simulink model "ASM_Traffic_V2X_Complete_Model_2"  (R2019a)
settings: Solver=ode1  StartTime=SIM.tstart.v  StopTime=Inf  FixedStep=SIM.StepSize.v  RelTol=1e-3
PostLoadFcn:
  | if any(exist('dsrtsu_mdlpostloadfcn', 'file') ~= 0), dsrtsu_mdlpostloadfcn('Execute', bdroot); end
  | try, asm_mdl_postloadfcn(bdroot, 'UpdateModel', 2200); catch, disp(lasterr); end,
undefined symbols (not defined in the file): _SensorPnts_1, _SensorPnts_13, _SensorPnts_17, _SensorPnts_21, _SensorPnts_25, _SensorPnts_29, _SensorPnts_33, _SensorPnts_37, _SensorPnts_41, _SensorPnts_45, _SensorPnts_49, _SensorPnts_5, _SensorPnts_53, _SensorPnts_57, _SensorPnts_9, _to_, CPT, G5A, ITS, MDL, rad, s_to_rpm, SIM
libraries: simulink x169, ASM_VehicleDynamics_lib x126, ASM_Traffic_lib x83, ASM_Utils_lib x49, mdbs x45, ASM_Environment_lib x17, dspindex x12, dsaV2xLibraryAux x10, dsmpblib x6, dsaV2xAsn1Library x4, dsaV2xLibrary x4, ASM_BrakeHydraulics_lib x4
(part 2 of 36)

== system ASM_Traffic_V2X_Complete_Model_2/MDL/SoftECU ==
  Vehicle_Signals : Inport
  Environment_Signals : Inport  Port=2
  ASMSignalCollector : Subsystem
  Bus Creator : BusCreator  Inputs=4
  Bus Creator1 : BusCreator  Inputs=5
  Bus Creator2 : BusCreator  Inputs=5
  Bus Creator3 : BusCreator  Inputs=6
  Bus Creator4 : BusCreator  Inputs=4
  Bus Creator5 : BusCreator  Inputs=1
  Bus Creator6 : BusCreator  Inputs=5
  Bus Selector : BusSelector  OutputSignals=Drivetrain.Transmission.ActiveTransmission.Gear[],Environment.Driver.OutputSignals.Pos_AccPedal[%],Environment.Driver.OutputSignals.AutomaticTrmCtrlSignals.SelectorLever[-3T|-2P|-1R|0N|1D],Environment.Driver.OutputSignals.AutomaticTrmCtrlSignals.SW_TipTronic[-1Down|0Off|1Up]
  Bus Selector1 : BusSelector  OutputSignals=Maneuver.Parameters.Gear_Max[],Maneuver.MdlControl.Reset_VehicleStates[0|1],Maneuver.RefSignals.Gear_Maneuver[],Maneuver.ModeSignals.GearClutch_Mode[1Stim|2Driver|3OpenClutch|4RefGear]
  Bus Selector10 : BusSelector  OutputSignals=VehicleDynamics.Steering.SteeringWheelTorque.TrqSensor_Steering[Nm]
  Bus Selector11 : BusSelector  OutputSignals=BasicEngine.EngineTorques.Trq_Eff_Engine[Nm],VehicleDynamics.Brake.MasterBrakeCylinder.ActiveBrakeCylinder.p[bar],VehicleDynamics.VehicleMovement.Velocities.Vehicle.Linear.v_Vehicle_CoG[x;y;z][km|h].v_x_Vehicle_CoG[km|h],VehicleDynamics.VehicleMovement.Velocities.Vehicle.Linear.v_Vehicle_CoG[x;y;z][km|h].v_y_Vehicle_CoG[km|h],VehicleDynamics.VehicleMovement.Accelerations.VehicleCoG.Linear.a_Vehicle_CoG[x;y;z][m|s2].a_y_Vehicle_CoG[m|s2],VehicleDynamics.VehicleMovement.Velocities.Vehicle.Angular.w_Vehicle_CoG[x;y;z][deg|s].YawRate_Vehicle_CoG[deg|s],VehicleDynamics.Wheel.WheelSpeed,VehicleDynamics.Steering.Angle_SteeringWheel[deg],VehicleDynamics.Steering.i_Steering_Mean[],Environment.Driver.OutputSignals.Pos_AccPedal[%],Environment.Driver.OutputSignals.Pos_BrakePedal[%],VehicleDynamics.Suspension.SuspensionRear.SuspensionKinematicsRear.Kinematics_Left.Position_Left.Pos_RL_Wheel[x;y;z][m],VehicleDynamics.Suspension.SuspensionFront.RelativePositionFront.Pos_Wheel[FL;FR][x;y;z][m].Pos_FL_Wheel[x;y;z][m]
  Bus Selector12 : BusSelector  OutputSignals=Drivetrain.Crankshaft.n_Engine[rad|s],Drivetrain.Transmission.AutomaticTransmission.GearBox.omega_In_Trm[rad|s],Drivetrain.Transmission.ActiveTransmission.omega_Out_Trm[rad|s]
  Bus Selector13 : BusSelector  OutputSignals=VehicleDynamics.Brake.BrakeDisc.Const_BrakeDiscFactor
  Bus Selector14 : BusSelector  OutputSignals=VehicleDynamics.Tire.Tire_FL.ActiveTire.r_Dyn_FL_Tire[m],VehicleDynamics.Tire.Tire_RL.ActiveTire.r_Dyn_RL_Tire[m],VehicleDynamics.Tire.Tire_FR.ActiveTire.r_Dyn_FR_Tire[m],VehicleDynamics.Tire.Tire_RR.ActiveTire.r_Dyn_RR_Tire[m]  OutputAsBus=on
  Bus Selector15 : BusSelector  OutputSignals=Environment.Driver.OutputSignals.StartButtonSignals.Sw_StartButton[0Off|1On],Environment.Driver.OutputSignals.AutomaticTrmCtrlSignals.SelectorLever[-3T|-2P|-1R|0N|1D],Environment.Driver.OutputSignals.Pos_BrakePedal[%],Environment.Driver.OutputSignals.Pos_ClutchPedal[%]
  Bus Selector16 : BusSelector  OutputSignals=Sw_Ignition[0|1],Sw_StarterReq[0|1]
  Bus Selector17 : BusSelector  OutputSignals=State_Engine[0|1|2|3|4]
  Bus Selector18 : BusSelector  OutputSignals=Factor_Trq_Engine_Red[%]
  Bus Selector19 : BusSelector  OutputSignals=State_Engine[0|1|2|3|4]
  Bus Selector2 : BusSelector  OutputSignals=ESP_Trq_Intervention.Enable_TrqIncrease_ESP[0|1],ESP_Trq_Intervention.Trq_IncreaseRequest_ESP[Nm],ESP_Trq_Intervention.Enable_TrqDecrease_Fast_ESP[0|1],ESP_Trq_Intervention.Trq_DecreaseRequest_Fast_ESP[Nm],ESP_Trq_Intervention.Enable_TrqDecrease_Slow_ESP[0|1],ESP_Trq_Intervention.Trq_DecreaseRequest_Slow_ESP[Nm]
  Bus Selector20 : BusSelector  OutputSignals=Sw_Ignition[0|1]
  Bus Selector21 : BusSelector  OutputSignals=Maneuver.MdlControl.Reset_VehicleStates[0|1]
  Bus Selector3 : BusSelector  OutputSignals=Drivetrain.Crankshaft.n_Engine[rpm],BasicEngine.EngineTorques.Trq_Driver_Des[Nm],Environment.Driver.OutputSignals.Pos_AccPedal[%]
  Bus Selector4 : BusSelector  OutputSignals=Maneuver.MdlControl.Reset_VehicleStates[0|1]
  Bus Selector5 : BusSelector  OutputSignals=Enable_Trq_Increase_ACC[0|1],Trq_IncreaseRequest_ACC[Nm]
  Bus Selector6 : BusSelector  OutputSignals=VehicleDynamics.VehicleMovement.Velocities.Vehicle.Linear.v_Vehicle_CoG[x;y;z][km|h]
  Bus Selector7 : BusSelector  OutputSignals=Maneuver.MdlControl.Reset_VehicleStates[0|1],Maneuver.UserSignals_Customized.ECU_Commands[]
  Bus Selector8 : BusSelector  OutputSignals=Enable_Trq_Decrease_ACC[0|1],Trq_DecreaseRequest_ACC[Nm]
  Bus Selector9 : BusSelector  OutputSignals=Maneuver.MdlControl.Reset_VehicleStates[0|1]
  DisableReset : Subsystem
      mask Display: disp('DisableReset')
  Map_Inputs : Subsystem
  ModelDesk_MC_ID_SoftECU : ASM_Utils_lib/ModelDeskInterface/ModelDesk_MC_ID_SoftECU  Tag=ASM_MAINCOMPONENT  ASMProperties=struct('Name','SoftECU')
  OpenBrkHydModel : Subsystem
      settings: OpenFcn=asm_open_lib('ASM_BrakeHydraulics_lib/Demos');
      mask Display: disp('Open\nASM_Brakehydraulics_lib')
  SOFT_ECU_POWERSTEERING : ASM_VehicleDynamics_lib/SoftECU/SoftECU_Steering/SOFT_ECU_POWERSTEERING  Tag=ASM_SUBCOMPONENT  Const_t_PowerSteering=MDL.SoftECU.SoftECUPowerSteering.Const_t_PowerSteering  Map_Trq_PowerSteering=MDL.SoftECU.SoftECUPowerSteering.Map_Trq_PowerSteering  StepSize=SIM.StepSize  ASMProperties=struct('Name','SOFT_ECU_POWERSTEERING','Version','3.0','Library','ASM_VehicleDynamics_lib')  ASMInstanceName=soft_ecu_powersteering  ASMInstanceID=1
  START_BUTTON : ASM_VehicleDynamics_lib/SoftECU/SoftECU_Body/START_BUTTON  Tag=ASM_SUBCOMPONENT  Const_t_Min_Active=MDL.SoftECU.StartButton.Const_t_Min_Active  Const_t_Min_Starter=MDL.SoftECU.StartButton.Const_t_Min_Starter  Const_Post_ClutchPedal_LowLim=MDL.SoftECU.StartButton.Const_Post_ClutchPedal_LowLim  Const_Post_BrakePedal_LowLim=MDL.SoftECU.StartButton.Const_Post_BrakePedal_LowLim  StepSize=SIM.StepSize  ASMProperties=struct('Name','START_BUTTON','Version','1.0','Library','ASM_VehicleDynamics_lib')  ASMInstanceName=start_button  ASMInstanceID=1
  Soft_ECU_ACC : Subsystem
  Soft_ECU_Brake : Subsystem  Tag=ASM_SOFT_ECU_BRAKE
      settings: AttributesFormatString=BASIC
  Soft_ECU_Engine_Basic : Subsystem
  Soft_ECU_Transmission : Subsystem
  StarterPermanentOn_Handling : Subsystem
  SoftECU_Signals : Outport
  tag scope: ASMBUS_SoftECU_ACC=global, ASMBUS_SoftECU_Brake=global, ASMBUS_SoftECU_Engine=global, ASMBUS_SoftECU_PowerSteering=global, ASMBUS_SoftECU_StartButton=global, ASMBUS_SoftECU_Transmission=global
  wires:
  DisableReset/1(Reset[0|1]) -> START_BUTTON/10
  Bus Selector21/1 -> DisableReset/1(Reset_VehicleStates[0|1])  "<Reset_VehicleStates[0|1]>"
  Bus Selector20/1 -> SOFT_ECU_POWERSTEERING/4  "<Sw_Ignition[0|1]>"
  Bus Selector19/1 -> Soft_ECU_Transmission/4(State_Engine[0|1|2|3|4])  "<State_Engine[0|1|2|3|4]>"
  [TAG_FromIO_Engine] -> Bus Selector17/1, Bus Selector19/1
  [TAG_FromIO_Drivetrain] -> Bus Selector18/1
  Bus Selector18/1 -> Soft_ECU_Engine_Basic/15(Factor_Trq_Engine_Red[%])  "<Factor_Trq_Engine_Red[%]>"
  Bus Selector16/2 -> Soft_ECU_Engine_Basic/5(Sw_StarterReq[0Off|1On])  "<Sw_StarterReq[0|1]>"
  Bus Selector16/1 -> Soft_ECU_Engine_Basic/4(Sw_Ignition[0Off|1On])  "<Sw_Ignition[0|1]>"
  [TAG_FromIO_Body] -> Bus Selector16/1, Bus Selector20/1
  START_BUTTON/1 -> [ASMBUS_SoftECU_StartButton]
  Bus Selector15/1 -> START_BUTTON/5  "<Sw_StartButton[0Off|1On]>"
  Bus Selector15/2 -> START_BUTTON/6  "<SelectorLever[-3T|-2P|-1R|0N|1D]>"
  Bus Selector15/3 -> START_BUTTON/7  "<Pos_BrakePedal[%]>"
  Bus Selector15/4 -> START_BUTTON/8  "<Pos_ClutchPedal[%]>"
  START_BUTTON/2 -> Bus Creator1/1  "State_StartButton[-2|-1|0|1|2|3]"
  START_BUTTON/6 -> Bus Creator1/5  "Sw_StarterReq[0|1]"
  START_BUTTON/3 -> Bus Creator1/2  "Lock[0|1]"
  START_BUTTON/4 -> Bus Creator1/3  "Sw_Acc[0|1]"
  START_BUTTON/5 -> Bus Creator1/4  "Sw_Ignition[0|1]"
  Bus Creator1/1 -> Bus Creator3/6  "ECU_Body"
  [TAG_Sw_Transmission_Mode] -> START_BUTTON/1
  [TAG_SoftECU_State_KeyFob] -> START_BUTTON/2
  Bus Selector17/1 -> START_BUTTON/9  "<State_Engine[0|1|2|3|4]>"
  StarterPermanentOn_Handling/1(State_StartButton_Ext[-1|0|1|2]) -> START_BUTTON/3
  StarterPermanentOn_Handling/2(Mode_StartButtonState[1Stim|2SoftECU]) -> START_BUTTON/4
  Bus Selector12/3 -> Soft_ECU_Transmission/3(omega_Out_Trm[rad|s])  "<omega_Out_Trm[rad|s]>"
  Bus Selector12/2 -> Soft_ECU_Transmission/2(omega_In_Trm[rad|s])  "<omega_In_Trm[rad|s]>"
  Bus Selector12/1 -> Soft_ECU_Transmission/1(n_Engine[rad|s])  "<n_Engine[rad|s]>"
  [TAG_SoftECU_ESP_Switches] -> Map_Inputs/3(Switches_ESP_User)
  Bus Selector7/2 -> Map_Inputs/2(ECU_Commands[])  "<ECU_Commands[]>"
  Map_Inputs/2(Sw_ASR[0Off|1On]) -> Soft_ECU_Brake/7(Sw_ASR[0Off|1On])
  Map_Inputs/1(Sw_ESP[0Off|1ABS|ESP]) -> Soft_ECU_Brake/6(Sw_ESP[0Off|1ABS|2ESP])
  Soft_ECU_Brake/1(ASMSignalBus) -> [ASMBUS_SoftECU_Brake]
  Soft_ECU_Brake/6(Trq_Intervention) -> Bus Creator6/5
  Soft_ECU_Brake/5(Valves) -> Bus Creator6/4
  Soft_ECU_Brake/4(ECU_Mode[0None|1ABS|2ESP|3ASR]) -> Bus Creator6/3
  Soft_ECU_Brake/3(p_Brake_Desired[bar]) -> Bus Creator6/2
  Soft_ECU_Brake/2(Enable_p_Brake_Desired[0|1]) -> Bus Creator6/1
  Bus Selector14/1 -> Soft_ECU_Brake/21(r_Tire[m])
  Bus Selector11/13 -> Soft_ECU_Brake/20(Pos_FL_Wheel[x;y;z][m])  "<Pos_FL_Wheel[x;y;z][m]>"
  Bus Selector11/12 -> Soft_ECU_Brake/19(Pos_RL_Wheel[x;y;z][m])  "<Pos_RL_Wheel[x;y;z][m]>"
  Bus Selector11/11 -> Soft_ECU_Brake/18(Pos_BrakePedal[%])  "<Pos_BrakePedal[%]>"
  Bus Selector11/10 -> Soft_ECU_Brake/17(Pos_AccPedal[%])  "<Pos_AccPedal[%]>"
  Bus Selector11/2 -> Soft_ECU_Brake/9(p_MasterBrakeCyl[bar])  "<p[bar]>"
  Bus Selector11/3 -> Soft_ECU_Brake/10(v_x_Vehicle_CoG[km|h])  "<v_x_Vehicle_CoG[km|h]>"
  Bus Selector11/4 -> Soft_ECU_Brake/11(v_y_Vehicle_CoG[km|h])  "<v_y_Vehicle_CoG[km|h]>"
  Bus Selector11/5 -> Soft_ECU_Brake/12(a_y_Vehicle_CoG[m|s2])  "<a_y_Vehicle_CoG[m|s2]>"
  Bus Selector11/6 -> Soft_ECU_Brake/13(YawRate_Vehicle_CoG[deg|s])  "<YawRate_Vehicle_CoG[deg|s]>"
  Bus Selector11/7 -> Soft_ECU_Brake/14(WheelSpeed[FL;FR;RL;RR][rad|s])  "<WheelSpeed>"
  Bus Selector11/8 -> Soft_ECU_Brake/15(Angle_SteeringWheel[deg])  "<Angle_SteeringWheel[deg]>"
  Bus Selector11/9 -> Soft_ECU_Brake/16(i_Steering_Mean[])  "<i_Steering_Mean[]>"
  Bus Selector11/1 -> Soft_ECU_Brake/8(Trq_Eff_Engine[Nm])  "<Trq_Eff_Engine[Nm]>"
  Bus Selector7/1 -> Soft_ECU_Brake/5(Reset[]), Map_Inputs/1(Reset[0|1])  "<Reset_VehicleStates[0|1]>"
  Bus Selector13/1 -> Soft_ECU_Brake/4(Const_BrakeDiscFactor[FL;FR;RL;RR][m3])  "<Const_BrakeDiscFactor>"
  Bus Selector9/1 -> SOFT_ECU_POWERSTEERING/2  "<Reset_VehicleStates[0|1]>"
  Bus Selector10/1 -> SOFT_ECU_POWERSTEERING/1  "<TrqSensor_Steering[Nm]>"
  Bus Selector/2 -> Soft_ECU_Transmission/6(Pos_AccPedal_Driver[%])  "<Pos_AccPedal[%]>"
  Bus Selector/3 -> Soft_ECU_Transmission/7(SelectorLever[-3T|-2P|-1R|0N|1D])  "<SelectorLever[-3T|-2P|-1R|0N|1D]>"
  Bus Selector/4 -> Soft_ECU_Transmission/8(TipShift[-1Down|0Off|1Up])  "<SW_TipTronic[-1Down|0Off|1Up]>"
  Bus Selector3/3 -> Soft_ECU_Engine_Basic/3(Pos_AccPedal_Driver[%])  "<Pos_AccPedal[%]>"
  Bus Selector8/2 -> Soft_ECU_Brake/3(Trq_Request_Extern[Nm])  "<Trq_DecreaseRequest_ACC[Nm]>"
  Bus Selector8/1 -> Soft_ECU_Brake/2(Enable_Trq_Extern[0|1]), Soft_ECU_Brake/1(State_Brake_Without_BrkPedal[0|1])  "<Enable_Trq_Decrease_ACC[0|1]>"
  Bus Selector1/2 -> Soft_ECU_Transmission/10(Reset[0|1])  "<Reset_VehicleStates[0|1]>"
  Bus Selector1/1 -> Soft_ECU_Transmission/9(Gear_Max_Maneuver[0Off|1_n])  "<Gear_Max[]>"
  Soft_ECU_Transmission/5(Gear[]) -> Bus Creator/4  "Gear[]"
  Soft_ECU_Transmission/4(Ctrl_Lockup_Clutch[%]) -> Bus Creator/3  "Ctrl_Lockup_Clutch[%]"
  Soft_ECU_Transmission/3(Ctrl_Parking_Pawl[0|1]) -> Bus Creator/2  "Ctrl_Parking_Pawl[0|1]"
  Soft_ECU_Transmission/1(ASMSignalBus) -> [ASMBUS_SoftECU_Transmission]
  Soft_ECU_Transmission/2(Factor_Trq_Engine_Red[%]) -> Bus Creator/1  "Factor_Trq_Engine_Red[%]"
  Bus Selector/1 -> Soft_ECU_Transmission/5(Gear_Current[])  "<Gear[]>"
  Bus Selector1/3 -> Soft_ECU_Transmission/11(Gear_Maneuver[])  "<Gear_Maneuver[]>"
  Bus Selector1/4 -> Soft_ECU_Transmission/12(GearClutch_Mode[1Stim|2SoftECU|3OpenClutch|4RefGear])  "<GearClutch_Mode[1Stim|2Driver|3OpenClutch|4RefGear]>"
  Bus Selector4/1 -> Soft_ECU_Engine_Basic/6(Reset[])  "<Reset_VehicleStates[0|1]>"
  Bus Selector3/1 -> Soft_ECU_Engine_Basic/1(n_Engine[rpm])  "<n_Engine[rpm]>"
  Bus Selector3/2 -> Soft_ECU_Engine_Basic/2(Trq_Driver_Des[Nm])  "<Trq_Driver_Des[Nm]>"
  Soft_ECU_Engine_Basic/2(Engine_Dynamic_Fast[0|1]) -> Bus Creator2/1  "Engine_Dynamic_Fast[0|1]"
  Soft_ECU_Engine_Basic/3(Pos_AccPedal_Influenced[%]) -> Bus Creator2/2  "Pos_AccPedal_Influenced[%]"
  Soft_ECU_Engine_Basic/4(Pos_AccPedal_Driver_Des[%]) -> Bus Creator2/3  "Pos_AccPedal_Driver_Des[%]"
  Bus Creator2/1 -> Bus Creator3/1  "ECU_Engine"
  Soft_ECU_Engine_Basic/1(ASMSignalBus) -> [ASMBUS_SoftECU_Engine]
  Soft_ECU_Engine_Basic/5(Sw_Starter[0Off|1On]) -> Bus Creator2/4  "Sw_Starter[0Off|1On]"
  Soft_ECU_Engine_Basic/6(State_Engine[0|1|2|3|4]) -> Bus Creator2/5  "State_Engine[0|1|2|3|4]"
  Bus Creator5/1 -> Bus Creator3/5  "ECU_PowerSteering"
  SOFT_ECU_POWERSTEERING/2 -> Bus Creator5/1  "Trq_PowerSteering[Nm]"
  Bus Selector6/1 -> SOFT_ECU_POWERSTEERING/3  "<v_Vehicle_CoG[x;y;z][km|h]>"
  SOFT_ECU_POWERSTEERING/1 -> [ASMBUS_SoftECU_PowerSteering]
  [TAG_FromIO_Brake] -> Bus Selector2/1
  Bus Selector2/1 -> Soft_ECU_Engine_Basic/7(Enable_TrqIncrease_Fast_ESP[0|1])  "<Enable_TrqIncrease_ESP[0|1]>"
  Bus Selector2/2 -> Soft_ECU_Engine_Basic/8(Trq_IncreaseRequest_Fast_ESP[Nm])  "<Trq_IncreaseRequest_ESP[Nm]>"
  Bus Selector2/3 -> Soft_ECU_Engine_Basic/9(Enable_TrqDecrease_Fast_ESP[0|1])  "<Enable_TrqDecrease_Fast_ESP[0|1]>"
  Bus Selector2/4 -> Soft_ECU_Engine_Basic/10(Trq_DecreaseRequest_Fast_ESP[Nm])  "<Trq_DecreaseRequest_Fast_ESP[Nm]>"
  Bus Selector2/5 -> Soft_ECU_Engine_Basic/11(Enable_TrqDecrease_Slow_ESP[0|1])  "<Enable_TrqDecrease_Slow_ESP[0|1]>"
  Bus Selector2/6 -> Soft_ECU_Engine_Basic/12(Trq_DecreaseRequest_Slow_ESP[Nm])  "<Trq_DecreaseRequest_Slow_ESP[Nm]>"
  Soft_ECU_ACC/2(Enable_Trq_Engine_ACC[0|1]) -> Bus Creator4/1  "Enable_Trq_Increase_ACC[0|1]"
  Soft_ECU_ACC/3(Trq_Request_Engine_ACC[Nm]) -> Bus Creator4/2  "Trq_IncreaseRequest_ACC[Nm]"
  Soft_ECU_ACC/4(Enable_Trq_Brake_ACC[0|1]) -> Bus Creator4/3  "Enable_Trq_Decrease_ACC[0|1]"
  Soft_ECU_ACC/5(Trq_Request_Brake_ACC[Nm]) -> Bus Creator4/4  "Trq_DecreaseRequest_ACC[Nm]"
  Bus Creator3/1 -> SoftECU_Signals/1  "SoftECU"
  Bus Creator6/1 -> Bus Creator3/3  "ECU_Brake"
  Bus Creator4/1 -> Bus Creator3/4  "ECU_ACC"
  Bus Creator/1 -> Bus Creator3/2  "ECU_Transmission"
  [TAG_FromIO_ACC] -> Bus Selector5/1, Bus Selector8/1
  Bus Selector5/1 -> Soft_ECU_Engine_Basic/13(Enable_Trq_Extern[0|1])  "<Enable_Trq_Increase_ACC[0|1]>"
  Bus Selector5/2 -> Soft_ECU_Engine_Basic/14(Trq_Request_Extern[Nm])  "<Trq_IncreaseRequest_ACC[Nm]>"
  Soft_ECU_ACC/1(ASMSignalBus) -> [ASMBUS_SoftECU_ACC]
  Vehicle_Signals/1 -> Bus Selector3/1, Bus Selector12/1, Bus Selector/1, Bus Selector13/1, Bus Selector11/1, Bus Selector14/1, Soft_ECU_ACC/2(Vehicle_Signals), Bus Selector10/1, Bus Selector6/1, Bus Selector15/1
  Environment_Signals/1 -> Bus Selector4/1, Bus Selector1/1, Bus Selector7/1, Soft_ECU_ACC/1(Environment_Signals), Bus Selector9/1, Bus Selector21/1

== system ASM_Traffic_V2X_Complete_Model_2/MDL/VehicleDynamics ==
  Trq_Shaft[FL,FR,RL,RR][Nm] : Inport
  Environment_Signals : Inport  Port=2
  AERODYNAMICS : ASM_VehicleDynamics_lib/VehicleDynamics/Aerodynamics/AERODYNAMICS  Tag=ASM_SUBCOMPONENT  Map_C_x=MDL.VehicleDynamics.Aerodynamics.Map_C_x  Map_C_y=MDL.VehicleDynamics.Aerodynamics.Map_C_y  Map_C_z=MDL.VehicleDynamics.Aerodynamics.Map_C_z  Map_C_M_x=MDL.VehicleDynamics.Aerodynamics.Map_C_M_x  Map_C_M_y=MDL.VehicleDynamics.Aerodynamics.Map_C_M_y  Map_C_M_z=MDL.VehicleDynamics.Aerodynamics.Map_C_M_z  Const_A_x=MDL.VehicleDynamics.Aerodynamics.Const_A_x  Const_PosVec_VtoRefAero=MDL.VehicleDynamics.Aerodynamics.Const_PosVec_RefAero_CoorSysV  Const_Char_Length=MDL.VehicleDynamics.Aerodynamics.Const_Char_Length  Const_Dens_Air=MDL.VehicleDynamics.Aerodynamics.Const_Dens_Air  ASMProperties=struct('Name','AERODYNAMICS','Version','5.0','Library','ASM_VehicleDynamics_lib')  ASMInstanceName=aerodynamics  ASMInstanceID=1
  ASMSignalCollector : Subsystem
  Brake : Subsystem
  Bus Selector1 : BusSelector  OutputSignals=Road.Road_ContactPoints.Sw_Tire_Parameter_Set_CP[FL;FR;RL;RR][1|2|3|4],Road.Road_ContactPoints.Fric_Coeff_CP[FL;FR;RL;RR][],Road.Road_ContactPoints.Pos_z_CP[FL;FR;RL;RR][m],Road.Road_ContactPoints.UnitVec_z_CP[FL;FR;RL;RR][x;y;z],Road.Road_InitialStates.Pos_Vehicle_Init_CoorSys_E[x;y;z][m],Road.Road_InitialStates.Angle_Vehicle_Init_CoorSys_E[x;y;z][rad],Maneuver.MdlControl.Reset_VehicleStates[0|1],Maneuver.MdlControl.Keep_VehiclePosition[0|1],Driver.Pos_BrakePedal[%],Driver.Angle_SteeringWheel[deg],Road.Road_ASMVeh.v_Wind_Coor_Sys_E[x;y;z][m|s],Road.Ambient.p_Ambient[Pa],Driver.ParkingBrakeSignals.Sw_ParkingBrake[0Off|1On],Road.Ambient.T_Ambient[degC],Driver.Pos_AccPedal[%],Maneuver.VehicleInitStates.q_dt_Vehicle_Init[6x1],Maneuver.RefSignals.Trq_Steering_Maneuver[Nm],Maneuver.RefSignals.Sw_SteeringMode_Maneuver[1Angle|2Trq]
  Bus Selector2 : BusSelector  OutputSignals=w_Rel_FL_Wheel_dDispl_SteeringRod_dt[x;y;z][rad|m],w_Rel_FR_Wheel_dDispl_SteeringRod_dt[x;y;z][rad|m]  OutputAsBus=on
  Bus Selector3 : BusSelector  OutputSignals=Pos_FL_Wheel_dDispl_SteeringRod[x;y;z][],Pos_FR_Wheel_dDispl_SteeringRod[x;y;z][]  OutputAsBus=on
  Bus Selector4 : BusSelector  OutputSignals=Trq_PowerSteering[Nm]  OutputAsBus=on
  Bus Selector5 : BusSelector  OutputSignals=EPSMotorStates_External[Angle;Angle_dt][rad;rad|s]  OutputAsBus=on
  CommonVehicleParameters : Subsystem
      settings: CopyFcn=|
      | try
      |  set_param(gcb,'LinkStatus', 'none')
      | catch
      | end
      mask Display: disp('Common vehicle parameters')
  Constant : Constant  Value=0
  DerivativeAddition : Subsystem
  F_External_CoorSys_V[x,y,z][N] : Constant  Value=[0 0 0]
  ModelDesk_MC_ID_VehicleDynamics : ASM_Utils_lib/ModelDeskInterface/ModelDesk_MC_ID_VehicleDynamics  Tag=ASM_MAINCOMPONENT  ASMProperties=struct('Name','VehicleDynamics')
  OR : Subsystem
  STEERING_3DOF_VARIABLE_RATIO : ASM_VehicleDynamics_lib/VehicleDynamics/Steering/STEERING_3DOF_VARIABLE_RATIO  Tag=ASM_SUBCOMPONENT  SW_EPSLocation=MDL.VehicleDynamics.Steering3DOF.SW_EPSLocation  SW_EPSSimulation=MDL.VehicleDynamics.Steering3DOF.SW_EPSSimulation  SW_ExternalEPSOutput=MDL.VehicleDynamics.Steering3DOF.SW_ExternalEPSOutput  SW_LocationColumnStiffness=MDL.VehicleDynamics.Steering3DOF.SW_LocationColumnStiffness  SW_DriverHand=MDL.VehicleDynamics.Steering3DOF.SW_DriverHand  Map_i_Steering=MDL.VehicleDynamics.Steering3DOF.Map_i_Steering  Const_i_EPSSteeringColumn=MDL.VehicleDynamics.Steering3DOF.Const_i_EPSSteeringColumn  Const_i_EPSSteeringRod=MDL.VehicleDynamics.Steering3DOF.Const_i_EPSSteeringRod  Const_Angle_Max_SteeringWheel=MDL.VehicleDynamics.Steering3DOF.Const_Angle_Max_SteeringWheel  Const_CardanAngle_UpperJoint=MDL.VehicleDynamics.Steering3DOF.Const_CardanAngle_UpperJoint  Const_CardanAngle_LowerJoint=MDL.VehicleDynamics.Steering3DOF.Const_CardanAngle_LowerJoint  Const_AngleOffsetCardanJoints=MDL.VehicleDynamics.Steering3DOF.Const_InitialAngle_LowerCardanJoint  Const_InitialAngle_UpperCardanJoint=MDL.VehicleDynamics.Steering3DOF.Const_InitialAngle_UpperCardanJoint  Const_MaxTorque_Driver=MDL.VehicleDynamics.Steering3DOF.Const_MaxTorque_Driver  Const_Inertia_SteeringWheel=MDL.VehicleDynamics.Steering3DOF.Const_Inertia_SteeringWheel  Const_Inertia_LowerSteeringColumn=MDL.VehicleDynamics.Steering3DOF.Const_Inertia_LowerSteeringColumn  SW_SteeringColumn_Stiffness=MDL.VehicleDynamics.Steering3DOF.SW_SteeringColumn_Stiffness  Map_TrqSpring_SteeringColumn=MDL.VehicleDynamics.Steering3DOF.Map_TrqSpring_SteeringColumn  Const_Stiffness_SteeringColumn=MDL.VehicleDynamics.Steering3DOF.Const_Stiffness_SteeringColumn  Const_Damping_SteeringColumn=MDL.VehicleDynamics.Steering3DOF.Const_Damping_SteeringColumn  Const_Time_SteeringWheel=MDL.VehicleDynamics.Steering3DOF.Const_Time_SteeringWheel  Const_Stiffness_DriverHand=MDL.VehicleDynamics.Steering3DOF.Const_Stiffness_DriverHand  Const_Damping_DriverHand=MDL.VehicleDynamics.Steering3DOF.Const_Damping_DriverHand  Const_Inertia_EPS=MDL.VehicleDynamics.Steering3DOF.Const_Inertia_EPS  Const_Stiffness_EPS=MDL.VehicleDynamics.Steering3DOF.Const_Stiffness_EPS  Const_Damping_EPS=MDL.VehicleDynamics.Steering3DOF.Const_Damping_EPS  Const_Damping_LowerSteeringColumn=MDL.VehicleDynamics.Steering3DOF.Const_Damping_LowerSteeringColumn  SW_SF_SteeringWheel=MDL.VehicleDynamics.Steering3DOF.SpringFriction.SW_SF_SteeringWheel  Const_Stiffness_SF_SteeringWheel=MDL.VehicleDynamics.Steering3DOF.SpringFriction.Const_Stiffness_SF_SteeringWheel  Const_LimitingTorque_SF_SteeringWheel=MDL.VehicleDynamics.Steering3DOF.SpringFriction.Const_LimitingTorque_SF_SteeringWheel  SW_ESF_SteeringWheel=MDL.VehicleDynamics.Steering3DOF.ExponentialSpringFriction.SW_ESF_SteeringWheel  Const_Stiffness_ESF_SteeringWheel=MDL.VehicleDynamics.Steering3DOF.ExponentialSpringFriction.Const_Stiffness_ESF_SteeringWheel  Const_LimitingTorque_ESF_SteeringWheel=MDL.VehicleDynamics.Steering3DOF.ExponentialSpringFriction.Const_LimitingTorque_ESF_SteeringWheel  SW_CF_SteeringRod=MDL.VehicleDynamics.Steering3DOF.CoulombFriction.SW_CF_SteeringRod  Const_LimitingForce_CF_SteeringRod=MDL.VehicleDynamics.Steering3DOF.CoulombFriction.Const_LimitingForce_CF_SteeringRod  Const_Damping_CF_SteeringRod=MDL.VehicleDynamics.Steering3DOF.CoulombFriction.Const_Damping_CF_SteeringRod  SW_MF_SteeringRod=MDL.VehicleDynamics.Steering3DOF.MaxwellFriction.SW_MF_SteeringRod  Const_Stiffness_MF_SteeringRod=MDL.VehicleDynamics.Steering3DOF.MaxwellFriction.Const_Stiffness_MF_SteeringRod  Const_LimitingForce_MF_SteeringRod=MDL.VehicleDynamics.Steering3DOF.MaxwellFriction.Const_LimitingForce_MF_SteeringRod  Const_Damping_MF_SteeringRod=MDL.VehicleDynamics.Steering3DOF.MaxwellFriction.Const_Damping_MF_SteeringRod  SW_SF_SteeringRod=MDL.VehicleDynamics.Steering3DOF.SpringFriction.SW_SF_SteeringRod  Const_Stiffness_SF_SteeringRod=MDL.VehicleDynamics.Steering3DOF.SpringFriction.Const_Stiffness_SF_SteeringRod  Const_LimitingForce_SF_SteeringRod=MDL.VehicleDynamics.Steering3DOF.SpringFriction.Const_LimitingForce_SF_SteeringRod  SW_ESF_SteeringRod=MDL.VehicleDynamics.Steering3DOF.ExponentialSpringFriction.SW_ESF_SteeringRod  Const_Stiffness_ESF_SteeringRod=MDL.VehicleDynamics.Steering3DOF.ExponentialSpringFriction.Const_Stiffness_ESF_SteeringRod  Const_LimitingForce_ESF_SteeringRod=MDL.VehicleDynamics.Steering3DOF.ExponentialSpringFriction.Const_LimitingForce_ESF_SteeringRod  StepSize=SIM.StepSize  ASMProperties=struct('Name','STEERING_3DOF_VARIABLE_RATIO','Version','8.0','Library','ASM_VehicleDynamics_lib')  ASMInstanceName=steering_3dof_variable_ratio  ASMInstanceID=1
  SignalSpecification : SignalSpecification  Dimensions=4
  Stabilization_F_External[3X6] : Constant  Value=zeros(3,6)
  Stabilization_Trq_External[3X6] : Constant  Value=zeros(3,6)
  Suspension : Subsystem
  Terminator{,1..3} (4 alike) : Terminator
  Tire : Subsystem
  Trq_External_CoorSys_V[x,y,z][Nm] : Constant  Value=[0 0 0]
  VehicleInits : Subsystem
  VehicleMovement : Subsystem
  WHEEL_SPEED : ASM_VehicleDynamics_lib/VehicleDynamics/WheelSpeed/WHEEL_SPEED  Tag=ASM_SUBCOMPONENT  StepSize=SIM.StepSize  ASMProperties=struct('Name','WHEEL_SPEED','Version','8.0','Library','ASM_VehicleDynamics_lib')  ASMInstanceName=wheel_speed  ASMInstanceID=1
  omega_Wheel[FL,FR,RL,RR][rad|s] : Outport
  tag scope: ASMBUS_VehicleDynamics_Aerodynamics=global, ASMBUS_VehicleDynamics_Brake=global, ASMBUS_VehicleDynamics_Steering=global, ASMBUS_VehicleDynamics_Suspension=global, ASMBUS_VehicleDynamics_Tire=global, ASMBUS_VehicleDynamics_VehicleMovement=global, ASMBUS_VehicleDynamics_WheelSpeed=global
  wires:
  Suspension/11(AirSuspensionSignals_Out) -> Terminator3/1
  Constant/1 -> Suspension/5(AirSuspensionSignals_In)
  [TAG_FromIO_Steering] -> Bus Selector5/1
  Bus Selector1/18 -> STEERING_3DOF_VARIABLE_RATIO/13  "<Sw_SteeringMode_Maneuver[1Angle|2Trq]>"
  Bus Selector1/17 -> STEERING_3DOF_VARIABLE_RATIO/12  "<Trq_Steering_Maneuver[Nm]>"
  Bus Selector3/1 -> STEERING_3DOF_VARIABLE_RATIO/2
  Bus Selector2/1 -> STEERING_3DOF_VARIABLE_RATIO/1
  STEERING_3DOF_VARIABLE_RATIO/3 -> Terminator1/1
  STEERING_3DOF_VARIABLE_RATIO/2 -> Terminator2/1
  Bus Selector4/1 -> STEERING_3DOF_VARIABLE_RATIO/14
  [TAG_FromIO_Steering] -> Bus Selector4/1
  Bus Selector5/1 -> STEERING_3DOF_VARIABLE_RATIO/11
  DerivativeAddition/1(SteeringWheel_Driver[Angle;Angle_dt][deg;deg|s]) -> STEERING_3DOF_VARIABLE_RATIO/6
  VehicleInits/2(q_dt_Init[:]) -> VehicleMovement/24(q_dt_Init[:])
  VehicleInits/3(q_Wheel_Init[:]) -> VehicleMovement/25(q_Wheel_Init[:])
  Bus Selector1/16 -> VehicleInits/1(q_dt_Vehicle_Init[6x1])  "<q_dt_Vehicle_Init[6x1]>"
  Bus Selector1/4 -> Tire/9(UnitVec_z_CP_CoorSys_E[FL,FR,RL,RR][x;y;z])  "<UnitVec_z_CP[FL;FR;RL;RR][x;y;z]>"
  Bus Selector1/3 -> Tire/8(" Pos_z_CP_CoorSys_E[FL,FR,RL,RR][m]")  "<Pos_z_CP[FL;FR;RL;RR][m]>"
  Bus Selector1/2 -> Tire/7(Coef_Fric_Road[FL,FR,RL,RR][])  "<Fric_Coeff_CP[FL;FR;RL;RR][]>"
  Bus Selector1/1 -> Tire/6(Sw_Tire_Parameter_Set[FL,FR,RL,RR][1|2|3|4])  "<Sw_Tire_Parameter_Set_CP[FL;FR;RL;RR][1|2|3|4]>"
  VehicleInits/1(omega_Wheel_Init[:][rad|s]) -> WHEEL_SPEED/6
  OR/1(Out) -> Tire/10(Reset[])
  Bus Selector1/8 -> OR/1(In1), VehicleMovement/15(KeepVehiclePosition[0|1])  "<Keep_VehiclePosition[0|1]>"
  Bus Selector1/15 -> Brake/7(Pos_AccPedal[%])  "<Pos_AccPedal[%]>"
  Bus Selector1/14 -> Brake/6(T_Ambient[degC])  "<T_Ambient[degC]>"
  STEERING_3DOF_VARIABLE_RATIO/4 -> Terminator/1
  Stabilization_Trq_External[3X6]/1 -> VehicleMovement/23(Stabilization_Trq_External[3X6])
  Stabilization_F_External[3X6]/1 -> VehicleMovement/22(Stabilization_F_External[3X6])
  Trq_External_CoorSys_V[x,y,z][Nm]/1 -> VehicleMovement/21(Trq_External_CoorSys_V[x,y,z][Nm])
  F_External_CoorSys_V[x,y,z][N]/1 -> VehicleMovement/20(F_External_CoorSys_V[x,y,z][N])
  Bus Selector1/13 -> Brake/5(Sw_ParkingBrake[0Off|1On])  "<Sw_ParkingBrake[0Off|1On]>"
  SignalSpecification/1 -> WHEEL_SPEED/2
  Bus Selector1/12 -> Brake/4(p_Ambient[Pa])  "<p_Ambient[Pa]>"
  Bus Selector1/10 -> DerivativeAddition/1(Angle_SteeringWheel_Driver[deg])  "<Angle_SteeringWheel[deg]>"
  Suspension/5(gRear_dq_Rear_dt[2x2][]) -> VehicleMovement/16(gRear_dq_Rear_dt[2x2][])
  Suspension/4(gFront_dq_Front_dt[2x2][]) -> VehicleMovement/17(gFront_dq_Front_dt[2x2][])
  Suspension/3(SuspensionKinematicRelations_Rear) -> VehicleMovement/18(SuspensionKinematicsRelations_Rear)
  Suspension/2(SuspensionKinematicRelations_Front) -> Bus Selector2/1, Bus Selector3/1, VehicleMovement/19(SuspensionKinematicsRelations_Front)
  VehicleMovement/11(q_Wheel[q1_Front;q2_Front;q1_Rear;q2_Rear][]) -> Suspension/1(q_Wheel[q1_Front;q2_Front;q1_Rear;q2_Rear][])
  VehicleMovement/10(q_Wheel_dt[q1_Front;q2_Front;q1_Rear;q2_Rear][]) -> Suspension/2(q_Wheel_dt[q1_Front;q2_Front;q1_Rear;q2_Rear][])
  Suspension/6(v_Rel_WheelBody[FL,FR,RL,RR][x;y;z][m|s]) -> VehicleMovement/11(v_Rel_WheelBody[FL,FR,RL,RR][x;y;z][m|s])
  Suspension/7(w_Rel_WheelBody[FL,FR,RL,RR][x;y;z][x;y;z][rad|s]) -> VehicleMovement/10(w_Rel_WheelBody[FL,FR,RL,RR][x y z][rad|s])
  Suspension/8(Pos_Wheels[FL,FR,RL,RR][x;y;z][m]) -> VehicleMovement/9(Pos_Wheel[FL,FR,RL,RR][x;y;z][m])
  Suspension/9(gF_Susp[q1_Front;q2_Front;q1_Rear;q2_Rear][]) -> VehicleMovement/8(gF_Susp[q1_Front;q2_Front;q1_Rear;q2_Rear][])
  WHEEL_SPEED/2 -> VehicleMovement/7(Trq_Shaft_CoorSys_V[FL,FR,RL,RR][x;y;z][Nm]), STEERING_3DOF_VARIABLE_RATIO/5
  WHEEL_SPEED/4 -> Tire/11(omega_Wheel[FL,FR,RL,RR][rad|s]), omega_Wheel[FL,FR,RL,RR][rad|s]/1
  Trq_Shaft[FL,FR,RL,RR][Nm]/1 -> SignalSpecification/1
  Tire/4(Stiffness_z_Tire[FL,FR,RL,RR][N|m]) -> VehicleMovement/5(Stiffness_z_Tire[FL,FR,RL,RR][N|m])
  Tire/1(ASMSignalBus) -> [ASMBUS_VehicleDynamics_Tire]
  Bus Selector1/5 -> VehicleMovement/12(Pos_Vehicle_Init_CoorSys_E[x;y;z][m])  "<Pos_Vehicle_Init_CoorSys_E[x;y;z][m]>"
  Bus Selector1/6 -> VehicleMovement/13(Angle_V_Init_CoorSys_E[x;y;z][rad])  "<Angle_Vehicle_Init_CoorSys_E[x;y;z][rad]>"
  [TAG_FromIO_Brake] -> Brake/3(IO_Signals)
  Suspension/10(UnitVec_y_Wheel_CoorSys_V[FL,FR,RL,RR][x;y;z]) -> WHEEL_SPEED/4, Tire/1(UnitVec_y_Wheel_CoorSys_V[FL,FR,RL,RR][x y z])
  VehicleMovement/9(F_Gravitational[FL,FR,RL,RR][x;y;z][N]) -> STEERING_3DOF_VARIABLE_RATIO/10
  Tire/5(Trq_Tire_Wheel[FL,FR,RL,RR][Nm]) -> WHEEL_SPEED/1
  VehicleMovement/7(F_Gyroscopic[FL,FR,RL,RR][x;y;z][N]) -> STEERING_3DOF_VARIABLE_RATIO/8
  VehicleMovement/8(Trq_Gyroscopic[FL,FR,RL,RR][x;y;z][Nm]) -> STEERING_3DOF_VARIABLE_RATIO/9
  Suspension/1(ASMSignalBus) -> [ASMBUS_VehicleDynamics_Suspension]
  Bus Selector1/11 -> AERODYNAMICS/3  "<v_Wind_Coor_Sys_E[x;y;z][m|s]>"
  Bus Selector1/9 -> Brake/2(Pos_BrakePedal[%])  "<Pos_BrakePedal[%]>"
  Bus Selector1/7 -> OR/2(In2), VehicleMovement/14(Reset[]), Suspension/6(Reset[]), STEERING_3DOF_VARIABLE_RATIO/7, Brake/1(Reset[]), WHEEL_SPEED/5  "<Reset_VehicleStates[0|1]>"
  Brake/2(Trq_Brake[FL,FR,RL,RR][Nm]) -> WHEEL_SPEED/3
  VehicleMovement/2(v_Abs_Vehicle_CoG[x;y;z][m|s]) -> AERODYNAMICS/2
  VehicleMovement/1(ASMSignalBus) -> [ASMBUS_VehicleDynamics_VehicleMovement]
  AERODYNAMICS/3 -> VehicleMovement/1(F_Aero_CoorSys_V[x;y;z][N])
  AERODYNAMICS/2 -> VehicleMovement/2(Trq_Aero_CoorSys_V[x;y;z][Nm])
  VehicleMovement/3(RotationMatrix_V_to_E_T[3x3]) -> AERODYNAMICS/1, Tire/2(RotationMatrix_V_to_E_T[3x3])
  VehicleMovement/6(w_Abs_Wheel_CoorSys_V[FL,FR,RL,RR][x,y,z][rad|s]) -> Tire/5(w_Abs_Wheel_CoorSys_V[FL,FR,RL,RR][x,y,z][rad|s])
  VehicleMovement/5(v_Abs_WheelBody_CoorSys_V[FL,FR,RL,RR][x y z][m|s]) -> Tire/4(v_Abs_WheelBody_CoorSys_V[FL,FR,RL,RR][x;y;z][m|s])
  VehicleMovement/4(Pos_Wheels_CoorSys_E[FL,FR,RL,RR][x;y;z][m]) -> Tire/3(Pos_Wheels_CoorSys_E[FL,FR,RL,RR][x,y,z][m])
  Tire/2(F_Tire_CoorSys_V[FL,FR,RL,RR][x;y;z][N]) -> VehicleMovement/3(F_Tire_CoorSys_V[FL,FR,RL,RR][x;y;z][N]), STEERING_3DOF_VARIABLE_RATIO/3, Suspension/3(F_Tire[FL;FR;RL;RR][x;y;z][N])
  STEERING_3DOF_VARIABLE_RATIO/1 -> [ASMBUS_VehicleDynamics_Steering]
  Tire/3(Trq_Tire_CoorSys_V[FL,FR,RL,RR][x;y;z][Nm]) -> STEERING_3DOF_VARIABLE_RATIO/4, Suspension/4(Trq_Tire[FL;FR;RL;RR][x;y;z][N|m]), VehicleMovement/4(Trq_Tire_CoorSys_V[FL,FR,RL,RR][x;y;z][Nm])
  WHEEL_SPEED/3 -> VehicleMovement/6(w_Wheel[FL,FR,RL,RR][x;y;z][rad|s])
  WHEEL_SPEED/1 -> [ASMBUS_VehicleDynamics_WheelSpeed]
  AERODYNAMICS/1 -> [ASMBUS_VehicleDynamics_Aerodynamics]
  Brake/1(ASMSignalBus) -> [ASMBUS_VehicleDynamics_Brake]
  Environment_Signals/1 -> Bus Selector1/1

== system ASM_Traffic_V2X_Complete_Model_2/MDLUserInterface/Drivetrain ==
  MDL_DISP : Subsystem
      mask Display: disp('Simulation results:\nArbitrary input to\nControlDesk from MDL')
  MDL_PAR : Subsystem
      mask Display: disp('Model parameters:\nContinuous output from\nControlDesk to MDL')
  MDL_TEST : Subsystem
      mask Display: disp('Simulation results:\nArbitrary input to\nWorkspace from MDL')
  ModelDesk_MC_ID_Drivetrain : ASM_Utils_lib/ModelDeskInterface/ModelDesk_MC_ID_Drivetrain  Tag=ASM_MAINCOMPONENT  ASMProperties=struct('Name','Drivetrain')

== system ASM_Traffic_V2X_Complete_Model_2/MDLUserInterface/Engine ==
  MDL_DISP : Subsystem
      mask Display: disp('Simulation results:\nArbitrary input to\nControlDesk from MDL')
  MDL_PAR : Subsystem
      mask Display: disp('Model parameters:\nContinuous output from\nControlDesk to MDL')
  MDL_TEST : Subsystem
      mask Display: disp('Simulation results:\nArbitrary input to\nWorkspace from MDL')
  ModelDesk_MC_ID_EngineBasic : ASM_Utils_lib/ModelDeskInterface/ModelDesk_MC_ID_EngineBasic  Tag=ASM_MAINCOMPONENT  ASMProperties=struct('Name','EngineBasic')

== system ASM_Traffic_V2X_Complete_Model_2/MDLUserInterface/Environment ==
  MDL_DISP : Subsystem
      mask Display: disp('Simulation results:\nArbitrary input to\nControlDesk from MDL')
  MDL_PAR : Subsystem
      mask Display: disp('Model parameters:\nContinuous output from\nControlDesk to MDL')
  MDL_TEST : Subsystem
      mask Display: disp('Simulation results:\nArbitrary input to\nWorkspace from MDL')
  ModelDesk_MC_ID_Environment : ASM_Utils_lib/ModelDeskInterface/ModelDesk_MC_ID_Environment  Tag=ASM_MAINCOMPONENT  ASMProperties=struct('Name','Environment')

== system ASM_Traffic_V2X_Complete_Model_2/MDLUserInterface/ModelDesk_Plotting ==
  ModelDesk_PlotSignalCollector : Subsystem  mask(MDLD_PLOT_COLLECTOR){}
      settings: OpenFcn=asm_mdld_plot_update_gui(gcb);
      settings: CopyFcn=|
      | try
      |  set_param(gcb,'LinkStatus', 'none')
      | catch
      | end
  wires:
  [ASMBUS_Complete] -> ModelDesk_PlotSignalCollector/1(ASMSignalBus)

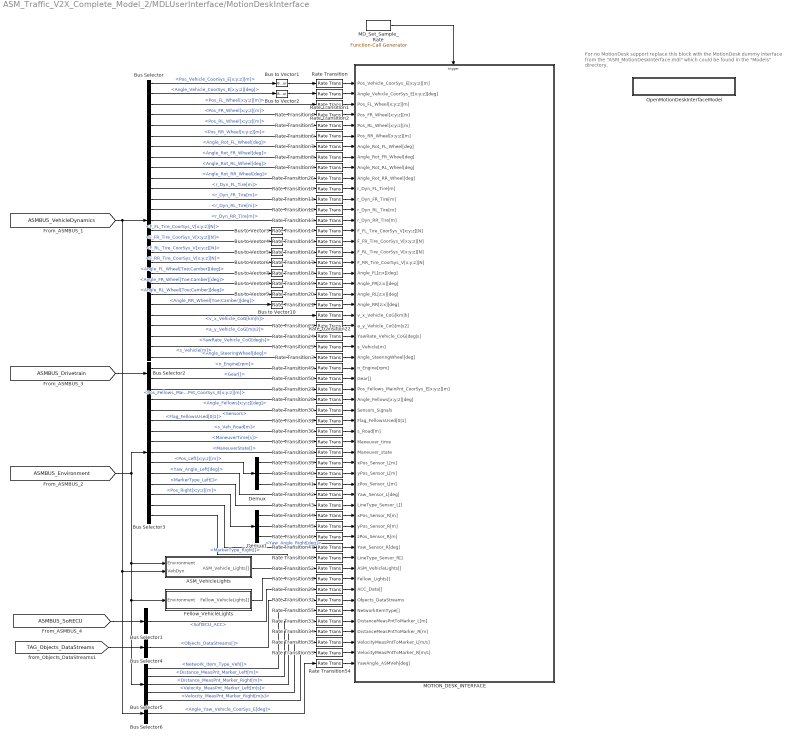
== system ASM_Traffic_V2X_Complete_Model_2/MDLUserInterface/MotionDeskInterface ==
  note: For no MotionDesk support replace this block  with the MotionDesk
      | dummy interface from the "ASM_MotionDeskInterface.mdl"
      | which could be found in the "Models" directory.
  ASM_VehicleLights : Subsystem
  Bus Selector : BusSelector  OutputSignals=VehicleMovement.Positions.Vehicle.Linear.Pos_Vehicle_CoorSys_E[x;y;z][m],VehicleMovement.Positions.Vehicle.Angular.Angle_Vehicle_CoorSys_E[x;y;z][deg],Suspension.SuspensionFront.RelativePositionFront.Pos_Wheel[FL;FR][x;y;z][m].Pos_FL_Wheel[x;y;z][m],Suspension.SuspensionFront.RelativePositionFront.Pos_Wheel[FL;FR][x;y;z][m].Pos_FR_Wheel[x;y;z][m],Suspension.SuspensionRear.RelativePositionRear.Pos_Wheel[RL;RR][x;y;z][m].Pos_RL_Wheel[x;y;z][m],Suspension.SuspensionRear.RelativePositionRear.Pos_Wheel[RL;RR][x;y;z][m].Pos_RR_Wheel[x;y;z][m],Wheel.RotationAngle.Angle_Rot_FL_Wheel[deg],Wheel.RotationAngle.Angle_Rot_FR_Wheel[deg],Wheel.RotationAngle.Angle_Rot_RL_Wheel[deg],Wheel.RotationAngle.Angle_Rot_RR_Wheel[deg],Tire.Tire_FL.ActiveTire.r_Dyn_FL_Tire[m],Tire.Tire_FR.ActiveTire.r_Dyn_FR_Tire[m],Tire.Tire_RL.ActiveTire.r_Dyn_RL_Tire[m],Tire.Tire_RR.ActiveTire.r_Dyn_RR_Tire[m],Tire.Tire_FL.TireForcesAndTorques.F_FL_Tire_CoorSys_V[x;y;z][N],Tire.Tire_FR.TireForcesAndTorques.F_FR_Tire_CoorSys_V[x;y;z][N],Tire.Tire_RL.TireForcesAndTorques.F_RL_Tire_CoorSys_V[x;y;z][N],Tire.Tire_RR.TireForcesAndTorques.F_RR_Tire_CoorSys_V[x;y;z][N],Suspension.SuspensionFront.RelativePositionFront.Angle_Wheel[FL;FR][Toe;Camber][deg].Angle_FL_Wheel[Toe;Camber][deg],Suspension.SuspensionFront.RelativePositionFront.Angle_Wheel[FL;FR][Toe;Camber][deg].Angle_FR_Wheel[Toe;Camber][deg],Suspension.SuspensionRear.RelativePositionRear.Angle_Wheel[RL;RR][Toe;Camber][deg].Angle_RL_Wheel[Toe;Camber][deg],Suspension.SuspensionRear.RelativePositionRear.Angle_Wheel[RL;RR][Toe;Camber][deg].Angle_RR_Wheel[Toe;Camber][deg],VehicleMovement.Velocities.Vehicle.Linear.v_Vehicle_CoG[x;y;z][km|h].v_x_Vehicle_CoG[km|h],VehicleMovement.Accelerations.VehicleCoG.Linear.a_Vehicle_CoG[x;y;z][m|s2].a_y_Vehicle_CoG[m|s2],VehicleMovement.Velocities.Vehicle.Angular.w_Vehicle_CoG[x;y;z][deg|s].YawRate_Vehicle_CoG[deg|s],VehicleMovement.Positions.Vehicle.Linear.s_Vehicle[m],Steering.Angle_SteeringWheel[deg]
  Bus Selector1 : BusSelector  OutputSignals=SoftECU_ACC
  Bus Selector2 : BusSelector  OutputSignals=Crankshaft.n_Engine[rpm],Transmission.ActiveTransmission.Gear[]
  Bus Selector3 : BusSelector  OutputSignals=Traffic.FellowMovement.FellowPositions.Pos_Fellows_MainPnt_CoorSys_E[x;y;z][m],Traffic.FellowMovement.FellowPositions.Angle_Fellows[x;y;z][deg],Traffic.Sensors,Traffic.FellowMovement.TrafficScheduler.Flag_FellowsUsed[0|1],Road.Road_ASMVeh.s_Veh_Road[m],Maneuver.ManeuverScheduler.Info.ManeuverTime[s],Maneuver.ManeuverScheduler.Info.ManeuverState[],Road.LaneSensor_Dynamic.Sensor_Output.CurrentLane.LeftSide.Pos_Left[x;y;z][m],Road.LaneSensor_Dynamic.Sensor_Output.CurrentLane.LeftSide.Yaw_Angle_Left[deg],Road.LaneSensor_Dynamic.Sensor_Output.CurrentLane.LeftSide.MarkerType_Left[],Road.LaneSensor_Dynamic.Sensor_Output.CurrentLane.RightSide.Pos_Right[x;y;z][m],Road.LaneSensor_Dynamic.Sensor_Output.CurrentLane.RightSide.Yaw_Angle_Right[deg],Road.LaneSensor_Dynamic.Sensor_Output.Lanes_Right.MarkerType_Right[]
  Bus Selector4 : BusSelector  OutputSignals=Objects_DataStreams[]
  Bus Selector5 : BusSelector  OutputSignals=Road.Road_Info.Network_Item_Type_Veh[],Road.LaneSensor_Dynamic.Sensor_Output.Measurement_Points.Distance_MeasPnt_Marker_Left[m],Road.LaneSensor_Dynamic.Sensor_Output.Measurement_Points.Distance_MeasPnt_Marker_Right[m],Road.LaneSensor_Dynamic.Sensor_Output.Measurement_Points.Velocity_MeasPnt_Marker_Left[m|s],Road.LaneSensor_Dynamic.Sensor_Output.Measurement_Points.Velocity_MeasPnt_Marker_Right[m|s]
  Bus Selector6 : BusSelector  OutputSignals=VehicleMovement.Positions.Vehicle.Angular.Angle_Vehicle_CoorSys_E[x;y;z][deg].Angle_Yaw_Vehicle_CoorSys_E[deg]
  Bus to Vector{1..10} (10 alike) : BusToVector
  Demux : Demux  Outputs=3
  Demux1 : Demux  Outputs=3
  Fellow_VehicleLights : Subsystem
  MD_Set_Sample_Rate : simulink/Ports & Subsystems/Function-Call Generator  sample_time=20*SIM.StepSize.v  numberOfIterations=1
  MOTION_DESK_INTERFACE : Subsystem
  OpenMotionDeskInterfaceModel : Subsystem
      settings: OpenFcn=|
      | InterfaceModel = 'ASM_MotionDeskInterface';
      | 
      | try
      |     open_system(InterfaceModel);                         catch
      |     errordlg(['ERROR opening MotionDesk interface: ',InterfaceModel,'.mdl.']);
      | end
      mask Display: disp('Open ASM_MotionDeskInterface')
  Rate Transition{,1..55} (56 alike) : RateTransition  Integrity=off  OutPortSampleTimeOpt=Inherit
  wires:
  Bus Selector5/1 -> Rate Transition55/1  "<Network_Item_Type_Veh[]>"
  Rate Transition55/1 -> MOTION_DESK_INTERFACE/51(NetworkItemType[])
  Rate Transition54/1 -> MOTION_DESK_INTERFACE/56(YawAngle_ASMVeh[deg])
  Rate Transition53/1 -> MOTION_DESK_INTERFACE/55(VelocityMeasPntToMarker_R[m/s])
  Rate Transition35/1 -> MOTION_DESK_INTERFACE/54(VelocityMeasPntToMarker_L[m/s])
  Rate Transition34/1 -> MOTION_DESK_INTERFACE/53(DistanceMeasPntToMarker_R[m])
  Rate Transition33/1 -> MOTION_DESK_INTERFACE/52(DistanceMeasPntToMarker_L[m])
  Bus Selector6/1 -> Rate Transition54/1  "<Angle_Yaw_Vehicle_CoorSys_E[deg]>"
  Bus Selector5/2 -> Rate Transition33/1  "<Distance_MeasPnt_Marker_Left[m]>"
  Bus Selector5/3 -> Rate Transition34/1  "<Distance_MeasPnt_Marker_Right[m]>"
  Bus Selector5/4 -> Rate Transition35/1  "<Velocity_MeasPnt_Marker_Left[m|s]>"
  Bus Selector5/5 -> Rate Transition53/1  "<Velocity_MeasPnt_Marker_Right[m|s]>"
  Bus Selector3/13 -> Rate Transition48/1  "<MarkerType_Right[]>"
  Bus Selector3/12 -> Rate Transition47/1  "<Yaw_Angle_Right[deg]>"
  Bus Selector3/11 -> Demux1/1  "<Pos_Right[x;y;z][m]>"
  Bus Selector3/10 -> Rate Transition43/1  "<MarkerType_Left[]>"
  Bus Selector3/9 -> Rate Transition42/1  "<Yaw_Angle_Left[deg]>"
  Bus Selector3/8 -> Demux/1  "<Pos_Left[x;y;z][m]>"
  Demux1/2 -> Rate Transition45/1
  Demux1/3 -> Rate Transition46/1
  Demux1/1 -> Rate Transition44/1
  Demux/2 -> Rate Transition40/1
  Demux/3 -> Rate Transition41/1
  Demux/1 -> Rate Transition39/1
  Bus to Vector7/1 -> Rate Transition18/1
  Bus to Vector8/1 -> Rate Transition19/1
  Bus to Vector9/1 -> Rate Transition20/1
  Bus to Vector10/1 -> Rate Transition21/1
  Bus to Vector6/1 -> Rate Transition17/1
  Bus to Vector5/1 -> Rate Transition16/1
  Bus to Vector4/1 -> Rate Transition15/1
  Bus to Vector3/1 -> Rate Transition14/1
  Bus to Vector2/1 -> Rate Transition1/1
  Bus to Vector1/1 -> Rate Transition/1
  Bus Selector/22 -> Bus to Vector10/1  "<Angle_RR_Wheel[Toe;Camber][deg]>"
  Bus Selector/21 -> Bus to Vector9/1  "<Angle_RL_Wheel[Toe;Camber][deg]>"
  Bus Selector/20 -> Bus to Vector8/1  "<Angle_FR_Wheel[Toe;Camber][deg]>"
  Bus Selector/19 -> Bus to Vector7/1  "<Angle_FL_Wheel[Toe;Camber][deg]>"
  Bus Selector/18 -> Bus to Vector6/1  "<F_RR_Tire_CoorSys_V[x;y;z][N]>"
  Bus Selector/17 -> Bus to Vector5/1  "<F_RL_Tire_CoorSys_V[x;y;z][N]>"
  Bus Selector/16 -> Bus to Vector4/1  "<F_FR_Tire_CoorSys_V[x;y;z][N]>"
  Bus Selector/15 -> Bus to Vector3/1  "<F_FL_Tire_CoorSys_V[x;y;z][N]>"
  Bus Selector/14 -> Rate Transition13/1  "<r_Dyn_RR_Tire[m]>"
  Bus Selector/13 -> Rate Transition12/1  "<r_Dyn_RL_Tire[m]>"
  Bus Selector/12 -> Rate Transition11/1  "<r_Dyn_FR_Tire[m]>"
  Bus Selector/11 -> Rate Transition10/1  "<r_Dyn_FL_Tire[m]>"
  Bus Selector/10 -> Rate Transition26/1  "<Angle_Rot_RR_Wheel[deg]>"
  Bus Selector/9 -> Rate Transition9/1  "<Angle_Rot_RL_Wheel[deg]>"
  Bus Selector/8 -> Rate Transition8/1  "<Angle_Rot_FR_Wheel[deg]>"
  Bus Selector/7 -> Rate Transition7/1  "<Angle_Rot_FL_Wheel[deg]>"
  Bus Selector/6 -> Rate Transition6/1  "<Pos_RR_Wheel[x;y;z][m]>"
  Bus Selector/5 -> Rate Transition5/1  "<Pos_RL_Wheel[x;y;z][m]>"
  Bus Selector/4 -> Rate Transition4/1  "<Pos_FR_Wheel[x;y;z][m]>"
  Bus Selector/3 -> Rate Transition2/1  "<Pos_FL_Wheel[x;y;z][m]>"
  Bus Selector/2 -> Bus to Vector2/1  "<Angle_Vehicle_CoorSys_E[x;y;z][deg]>"
  Bus Selector/1 -> Bus to Vector1/1  "<Pos_Vehicle_CoorSys_E[x;y;z][m]>"
  Bus Selector/27 -> Rate Transition3/1  "<Angle_SteeringWheel[deg]>"
  [ASMBUS_VehicleDynamics] -> ASM_VehicleLights/2(VehDyn), Bus Selector6/1, Bus Selector/1
  Bus Selector/23 -> Rate Transition22/1  "<v_x_Vehicle_CoG[km|h]>"
  Bus Selector/24 -> Rate Transition23/1  "<a_y_Vehicle_CoG[m|s2]>"
  Bus Selector/25 -> Rate Transition24/1  "<YawRate_Vehicle_CoG[deg|s]>"
  Bus Selector/26 -> Rate Transition25/1  "<s_Vehicle[m]>"
  Rate Transition/1 -> MOTION_DESK_INTERFACE/1(Pos_Vehicle_CoorSys_E[x;y;z][m])
  Rate Transition1/1 -> MOTION_DESK_INTERFACE/2(Angle_Vehicle_CoorSys_E[x;y;z][deg])
  Rate Transition2/1 -> MOTION_DESK_INTERFACE/3(Pos_FL_Wheel[x;y;z][m])
  Rate Transition4/1 -> MOTION_DESK_INTERFACE/4(Pos_FR_Wheel[x;y;z][m])
  Rate Transition5/1 -> MOTION_DESK_INTERFACE/5(Pos_RL_Wheel[x;y;z][m])
  Rate Transition6/1 -> MOTION_DESK_INTERFACE/6(Pos_RR_Wheel[x;y;z][m])
  Rate Transition7/1 -> MOTION_DESK_INTERFACE/7(Angle_Rot_FL_Wheel[deg])
  Rate Transition8/1 -> MOTION_DESK_INTERFACE/8(Angle_Rot_FR_Wheel[deg])
  Rate Transition9/1 -> MOTION_DESK_INTERFACE/9(Angle_Rot_RL_Wheel[deg])
  Rate Transition26/1 -> MOTION_DESK_INTERFACE/10(Angle_Rot_RR_Wheel[deg])
  Rate Transition10/1 -> MOTION_DESK_INTERFACE/11(r_Dyn_FL_Tire[m])
  Rate Transition11/1 -> MOTION_DESK_INTERFACE/12(r_Dyn_FR_Tire[m])
  Rate Transition12/1 -> MOTION_DESK_INTERFACE/13(r_Dyn_RL_Tire[m])
  Rate Transition13/1 -> MOTION_DESK_INTERFACE/14(r_Dyn_RR_Tire[m])
  Rate Transition14/1 -> MOTION_DESK_INTERFACE/15(F_FL_Tire_CoorSys_V[x;y;z][N])
  Rate Transition15/1 -> MOTION_DESK_INTERFACE/16(F_FR_Tire_CoorSys_V[x;y;z][N])
  Rate Transition16/1 -> MOTION_DESK_INTERFACE/17(F_RL_Tire_CoorSys_V[x;y;z][N])
  Rate Transition17/1 -> MOTION_DESK_INTERFACE/18(F_RR_Tire_CoorSys_V[x;y;z][N])
  Rate Transition18/1 -> MOTION_DESK_INTERFACE/19(Angle_FL[z;x][deg])
  Rate Transition19/1 -> MOTION_DESK_INTERFACE/20(Angle_FR[z;x][deg])
  Rate Transition20/1 -> MOTION_DESK_INTERFACE/21(Angle_RL[z;x][deg])
  Rate Transition21/1 -> MOTION_DESK_INTERFACE/22(Angle_RR[z;x][deg])
  Rate Transition22/1 -> MOTION_DESK_INTERFACE/23(v_x_Vehicle_CoG[km|h])
  Rate Transition23/1 -> MOTION_DESK_INTERFACE/24(a_y_Vehicle_CoG[m|s2])
  Rate Transition24/1 -> MOTION_DESK_INTERFACE/25(YawRate_Vehicle_CoG[deg|s])
  Rate Transition25/1 -> MOTION_DESK_INTERFACE/26(s_Vehicle[m])
  Rate Transition3/1 -> MOTION_DESK_INTERFACE/27(Angle_SteeringWheel[deg])
  Bus Selector4/1 -> Rate Transition32/1  "<Objects_DataStreams[]>"
  Rate Transition32/1 -> MOTION_DESK_INTERFACE/50(Objects_DataStreams)
  [TAG_Objects_DataStreams] -> Bus Selector4/1
  Rate Transition29/1 -> MOTION_DESK_INTERFACE/49(ACC_Data[])
  Bus Selector1/1 -> Rate Transition29/1  "<SoftECU_ACC>"
  [ASMBUS_SoftECU] -> Bus Selector1/1
  Rate Transition48/1 -> MOTION_DESK_INTERFACE/46(LineType_Sensor_R[])
  Rate Transition47/1 -> MOTION_DESK_INTERFACE/45(Yaw_Sensor_R[deg])
  Rate Transition46/1 -> MOTION_DESK_INTERFACE/44(zPos_Sensor_R[m])
  Rate Transition45/1 -> MOTION_DESK_INTERFACE/43(yPos_Sensor_R[m])
  Rate Transition44/1 -> MOTION_DESK_INTERFACE/42(xPos_Sensor_R[m])
  Rate Transition43/1 -> MOTION_DESK_INTERFACE/41(LineType_Sensor_L[])
  Rate Transition42/1 -> MOTION_DESK_INTERFACE/40(Yaw_Sensor_L[deg])
  Rate Transition41/1 -> MOTION_DESK_INTERFACE/39(zPos_Sensor_L[m])
  Rate Transition40/1 -> MOTION_DESK_INTERFACE/38(yPos_Sensor_L[m])
  Rate Transition39/1 -> MOTION_DESK_INTERFACE/37(xPos_Sensor_L[m])
  Rate Transition38/1 -> MOTION_DESK_INTERFACE/36(Maneuver_state)
  Bus Selector3/7 -> Rate Transition38/1  "<ManeuverState[]>"
  Bus Selector3/6 -> Rate Transition37/1  "<ManeuverTime[s]>"
  Bus Selector3/5 -> Rate Transition36/1  "<s_Veh_Road[m]>"
  Bus Selector2/2 -> Rate Transition50/1  "<Gear[]>"
  Bus Selector2/1 -> Rate Transition49/1  "<n_Engine[rpm]>"
  [ASMBUS_Drivetrain] -> Bus Selector2/1
  [ASMBUS_Environment] -> Bus Selector3/1, Bus Selector5/1, Fellow_VehicleLights/1(Environment), ASM_VehicleLights/1(Environment)
  MD_Set_Sample_Rate/1 -> MOTION_DESK_INTERFACE/Trigger
  Bus Selector3/1 -> Rate Transition27/1  "<Pos_Fellows_MainPnt_CoorSys_E[x;y;z][m]>"
  Bus Selector3/2 -> Rate Transition28/1  "<Angle_Fellows[x;y;z][deg]>"
  Bus Selector3/3 -> Rate Transition30/1  "<Sensors>"
  Bus Selector3/4 -> Rate Transition31/1  "<Flag_FellowsUsed[0|1]>"
  Rate Transition27/1 -> MOTION_DESK_INTERFACE/30(Pos_Fellows_MainPnt_CoorSys_E[x;y;z][m])
  Rate Transition28/1 -> MOTION_DESK_INTERFACE/31(Angle_Fellows[x;y;z][deg])
  Rate Transition30/1 -> MOTION_DESK_INTERFACE/32(Sensors_Signals)
  Rate Transition31/1 -> MOTION_DESK_INTERFACE/33(Flag_FellowsUsed[0|1])
  Rate Transition36/1 -> MOTION_DESK_INTERFACE/34(s_Road[m])
  Rate Transition37/1 -> MOTION_DESK_INTERFACE/35(Maneuver_time)
  Rate Transition49/1 -> MOTION_DESK_INTERFACE/28(n_Engine[rpm])
  Rate Transition50/1 -> MOTION_DESK_INTERFACE/29(Gear[])
  ASM_VehicleLights/1(ASM_Vehicle_Lights[]) -> Rate Transition52/1
  Fellow_VehicleLights/1(Fellow_VehicleLights[]) -> Rate Transition51/1
  Rate Transition51/1 -> MOTION_DESK_INTERFACE/48(Fellow_Lights[])
  Rate Transition52/1 -> MOTION_DESK_INTERFACE/47(ASM_VehicleLights[])

== system ASM_Traffic_V2X_Complete_Model_2/MDLUserInterface/OpenMotionDeskInterfaceModel ==

== system ASM_Traffic_V2X_Complete_Model_2/MDLUserInterface/SoftECU ==
  MDL_DISP : Subsystem
      mask Display: disp('Simulation results:\nArbitrary input to\nControlDesk from MDL')
  MDL_PAR : Subsystem
      mask Display: disp('Model parameters:\nContinuous output from\nControlDesk to MDL')
  MDL_TEST : Subsystem
      mask Display: disp('Simulation results:\nArbitrary input to\nWorkspace from MDL')
  ModelDesk_MC_ID_SoftECU : ASM_Utils_lib/ModelDeskInterface/ModelDesk_MC_ID_SoftECU  Tag=ASM_MAINCOMPONENT  ASMProperties=struct('Name','SoftECU')

== system ASM_Traffic_V2X_Complete_Model_2/MDLUserInterface/VehicleDynamics ==
  MDL_DISP : Subsystem
      mask Display: disp('Simulation results:\nArbitrary input to\nControlDesk from MDL')
  MDL_PAR : Subsystem
      mask Display: disp('Model parameters:\nContinuous output from\nControlDesk to MDL')
  MDL_TEST : Subsystem
      mask Display: disp('Simulation results:\nArbitrary input to\nWorkspace from MDL')
  ModelDesk_MC_ID_VehicleDynamics : ASM_Utils_lib/ModelDeskInterface/ModelDesk_MC_ID_VehicleDynamics  Tag=ASM_MAINCOMPONENT  ASMProperties=struct('Name','VehicleDynamics')

== system ASM_Traffic_V2X_Complete_Model_2/IO/I//O_Subsystem/Bus Configuration (1) - In ==
  Input : Inport
  Simulated ECUs : Subsystem
  _In_ : BusCreator  Inputs=1
  In : Outport
  wires:
  _In_/1 -> In/1  "In"
  Simulated ECUs/1(Simulated ECUs) -> _In_/1  "Simulated ECUs"
  Input/1 -> Simulated ECUs/1(Input)

== system ASM_Traffic_V2X_Complete_Model_2/IO/I//O_Subsystem/Bus Configuration (1) - Out ==
  Out : Inport
  Simulated ECUs : Subsystem
  _Out_ : BusSelector  OutputSignals=Simulated ECUs
  wires:
  Out/1 -> _Out_/1  "Out"
  _Out_/1 -> Simulated ECUs/1(Simulated ECUs)  "<Simulated ECUs>"
